simulink library "DBX_Control_lib"  (R2015a)
settings: Solver=ode45  SolverMode=SingleTasking  StartTime=0.0  StopTime=10.0  RelTol=1e-3
undefined symbols (not defined in the file or in its folder): a, A_M, C_d0, CG, h_1, h_2, h_3, kappa_Q, kappa_T, L_M, lambda_0_Q, lambda_0_T, m, Newton, Omega_TO, R, Raphson, rho, Rotation_sign, sigma, T_ctrl, theta_0, theta_1, Throtle_TO, Throtle_TTO_vec, v_i0, v_i_adim, Vx_adim, Vz_adim
undefined symbols (not defined in the file): hp_1, T_sim
libraries: DBX_Control_lib x15, simulink x8, vrlib x7, DBX_model x3, qcatlib x1, XXCopter_Control x1
(part 1 of 2)
settings Model: Creator=David  LastModifiedBy=David
settings OptimizationCC: BlockReduction=off  BooleanDataType=off
settings DebuggingCC: SaveWithParameterizedLinksMsg=none  UnderspecifiedInitializationDetection=Classic  MergeDetectMultiDrivingBlocksExec=none  SignalResolutionControl=TryResolveAllWithWarning  StrictBusMsg=Warning
settings HardwareCC: TargetUnknown=on

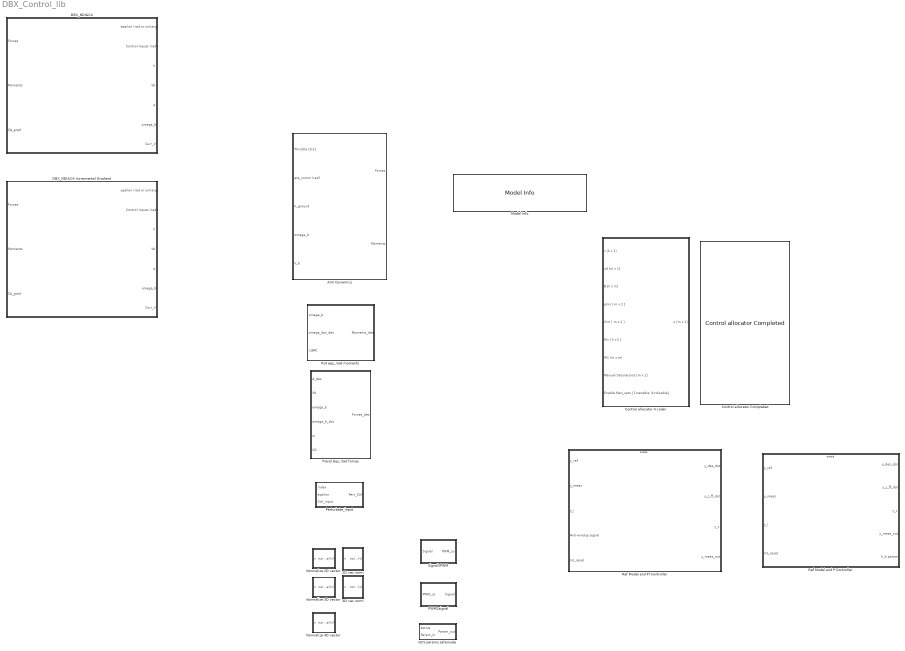
== system DBX_Control_lib ==
  2D vec norm : Subsystem  TreatAsAtomicUnit=on
  3D vec norm : Subsystem  TreatAsAtomicUnit=on
  Arm Dynamics : Subsystem  TreatAsAtomicUnit=on  mask(Arm dynamics, kinematics, forces and moments){arm_num=1, Rot_sign=Rotation_sign(1), Hub_pos=[1/3*L_M;-A_M/2;h_1], h_p=hp_1}
      mask prompts: arm_num "Arm number (1,2 or 3)"; Rot_sign "Rotation Sign"; Hub_pos "Hub position"; h_p "Hub to porpeller dist"
      mask help:
      | This block only accepts arms oriented in x-axis or y-axis: eta direction can only be [1,0,0] or [0,1,0]
      |
      | If Arm number 1 or  2 (Forward ones)
      | eta_dir==[0,1,0]
      |
      | If Arm number 3 (rear one)
      | eta_dir=[1,0,0]
      |
      | Usar SIEMPRE SI
      mask TypeOptions arm_num: Arms Kinematics DBX/Value
      mask TypeOptions Rot_sign: Aerodynamics Propeller DBX/Rot_signa
      mask TypeOptions Hub_pos: Arms Kinematics DBX/Hub_pos
      mask TypeOptions h_p: Arms Kinematics DBX/h_p
      mask DialogControl ParameterTabVar0 Prompt: Arm parameters
      mask Display: disp(['{\bf \fontsize{16}',sprintf('Arm number\n\n'),num2str(arm_num),sprintf('\n\n Dynamics '),'}'], 'texmode','on');
  Control allocator 4 coder : Subsystem  mask(Control allocator WLS){gamma=1e6, imax=100, T=T_sim}
      mask prompts: gamma "Weight of Control Error Cost (gamma)"; imax "Max # of iterations"; T "Sample Time"
      mask help:
      | Author: David Torres
      | Based on work of Ola Härkegård
  "Control allocator Completed " : qcatlib/Control allocator Completed   alg=WLS  CA_type=QP  iter_max=100  gamma=1  k_B=6  m_B=9  T=T_ctrl  tol=1e-5
  DBX_NDI&CA : Subsystem  TreatAsAtomicUnit=on
  DBX_NDI&CA Incremental Gradient : Subsystem  TreatAsAtomicUnit=on
  GCS params safemode : Subsystem  TreatAsAtomicUnit=on
  Model Info : simulink/Model-Wide Utilities/Model Info  Frame=on  DisplayStringWithTags=|  HorizontalTextAlignment=Center  LeftAlignmentValue=0.5  SourceBlockDiagram=DBX_Control_lib  TagMaxNumber=20
      | Model Info
      | 
      | Creado por %<Creator>
      | Modificado el %<LastModificationDate> por %<LastModifiedBy>
      | Version %<ModelVersion>
  Normalize 2D vector : Subsystem  TreatAsAtomicUnit=on
  Normalize 3D vector : Subsystem  TreatAsAtomicUnit=on
  Normalize 4D vector : Subsystem  TreatAsAtomicUnit=on
  PWM2signal : Subsystem  TreatAsAtomicUnit=on  mask{c=2100, a=900, d=1, b=0}
      mask prompts: c "PWM sup limit (us)"; a "PWM inf limit (us)"; d "Signal sup limit"; b "Signal inf limit"
      mask TypeOptions c: up_PWM/Value
      mask TypeOptions a: down_PWM/Value
      mask TypeOptions d: up_signal/Value
      mask TypeOptions b: down_signal/Value
  Perturbate_input : Subsystem
  Ref Model and P Controller : Subsystem  mask(Reference Model and Controller){tau=0.2, RisingSlewLimit=4, FallingSlewLimit=-4, K_f=1, K_b=1}
      mask prompts: tau "Desired time constant tau"; RisingSlewLimit "Reference max rising rate"; FallingSlewLimit "Reference max falling rate"; K_f "Rate Feedfordward Gain K_f"; K_b "Proportional Gain K_b"
      mask help:
      | Author: David Torres
      |
      | This block allows a design of the desired dynamics as a 1st order system and the controller of it with P and I actions, with feedforward in rate and anti-windup action.
      |
      |     Inputs: Signal reference, Signal measurement and anti-windup dignal.
      |     Outputs: Desired Signal rate
      |
      | The block shows the expected dynamics assuming the output is integrated with a PERFECT INTEGRATOR or an INTEGRATOR WITH DELAY(delta):
      |      NDI, CA and plant act as a perfect integrator or integrator with a delay delta.
      mask TypeOptions tau: Reference Model/tau
      mask TypeOptions RisingSlewLimit: Rate Limiter/RisingSlewLimit
      mask TypeOptions FallingSlewLimit: Rate Limiter/FallingSlewLimit
      mask TypeOptions K_f: K_f/Gain
      mask TypeOptions K_b: K_b params/Value
      mask Display:
      | K_ref=1/tau;
      | TF = tf([K_ref],[1 K_ref]);
      | 
      | [y,t]=step(TF);
      | S = stepinfo(y,t);
      | 
      | pos = get_param(gcb, 'Position');
      | width = pos(3) - pos(1);
      | height = pos(4) - pos(2);
      | t = t.*width/max(t);
      | y=y.*height/max(y);
      | plot(t,y);
      | S2 = stepinfo(y,t);
      | 
      | if S.Overshoot==0 % 1st order response
      |     text(S2.RiseTime ,height*0.85,['Rise time = ',num2str(S.RiseTime),'s' ]);
      |     text(S2.RiseTime ,height*0.75,['Settling Time = ',num2str(S.SettlingTime)]);
      | 
      | elseif S.Overshoot<0.05 % 2nd order response
      |     text(width*0.5 ,height*0.9,['Rise time = ',num2str(S.RiseTime),'s' ]);
      |     text(width*0.5 ,height*0.8,['Pike time = ',num2str(S.PeakTime),'s' ]);
      |     text(width*0.5 ,height*0.7,['Os = ',num2str(S.Peak)]);
      |     text(width*0.5 ,height*0.6,['SettlingTime = ',num2str(S.SettlingTime)]);
      | else % 2nd order response
      |     text(S2.PeakTime ,S2.Peak*0.85,['Peak time = ',num2str(S.PeakTime),'s' ]);
      |     text(S2.PeakTime ,S2.Peak*0.75,['Os = ',num2str(S.Peak)]);
      |     text(S2.PeakTime ,S2.Peak*0.65,['SettlingTime = ',num2str(S.SettlingTime)]);
      | end
      | 
      | 
      | [num,den] = tfdata(TF);
      | dpoly(num{:},den{:}, 's');
  Ref Model and PI Controller : Subsystem  mask(Reference Model and Controller){delta=0, tau=0.5, RisingSlewLimit=4, FallingSlewLimit=-4, K_f=1, K_a=1, Con_way=pro, omega_n=4, xi=0.5, Z1=-30, K_b=2*0.8*3, f_i=0.25*1/0.8^2, f_c=1}
      mask prompts: delta "Delay on assumed integration: delta (0 for ideal integration)"; tau "Desired time constant tau"; RisingSlewLimit "Reference max rising rate"; FallingSlewLimit "Reference max falling rate"; K_f "Rate Feedfordward Gain"; K_a "Anti-windup gain K_a"; Con_way "Expected response: Controller Design process"; omega_n "Desired 2nd order response omega_n"; xi "Desired 2nd order response  xi"; Z1 "Zero of controller"
      mask help:
      | Author: David Torres
      |
      | This block allows a design of the desired dynamics as a 1st order system and the controller of it with P and I actions, with feedforward in rate and anti-windup action.
      |
      |     Inputs: Signal reference, Signal measurement and anti-windup dignal.
      |     Outputs: Desired Signal rate
      |
      | The block shows the expected dynamics assuming the output is integrated with a PERFECT INTEGRATOR or an INTEGRATOR WITH DELAY(delta):
      |      NDI, CA and plant act as a perfect integrator or integrator with a delay delta.
      mask init:
      | val = get_param(gcb,'MaskValues');
      | 
      | K_ref=1/tau;	
      | % Controller design
      | switch lower(char(val{7}))
      |     case 'auto'
      |         K_b=2*xi*omega_n
      |         f_i=1/(4*xi^2)
      |         if f_i<0.25
      |             f_c = 0.5*(1+sqrt(1-4*f_i));
      |         else
      |             f_c = sqrt(f_i);
      |         end
      |         f_c
      |     case 'advanced'
      |         K_b=2*xi*omega_n;
      |         f_i=1/(4*xi^2);
      |         f_c =  -omega_n/(2*xi*Z1);  
      |     case 'pro'
      | end
      mask TypeOptions delta: PI Controller/delta
      mask TypeOptions tau: Reference Model/tau
      mask TypeOptions RisingSlewLimit: Rate Limiter/RisingSlewLimit
      mask TypeOptions FallingSlewLimit: Rate Limiter/FallingSlewLimit
      mask TypeOptions K_f: K_f/Gain
      mask TypeOptions K_a: PI Controller/K_a
      mask TypeOptions Con_way: auto | advanced | pro
      mask Callback Con_way:
      | val = get_param(gcb,'MaskValues');
      | switch lower(char(val{7}))
      |  case 'auto'
      |      set_param(gcb,'MaskVisibilities',{'on','on','on','on','on','on','on','on','on','off','off','off','off'});
      |  case 'advanced'
      |      set_param(gcb,'MaskVisibilities',{'on','on','on','on','on','on','on','on','on','on','off','off','off'});
      |  case 'pro'
      |      set_param(gcb,'MaskVisibilities',{'on','on','on','on','on','on','on','off','off','off','on','on','on'});
      |  end
      mask TypeOptions K_b: PI Controller/K_b
      mask TypeOptions f_i: PI Controller/f_i
      mask TypeOptions f_c: PI Controller/f_c
      mask Display:
      | RM = tf([K_ref],[1 K_ref]);
      | 
      | if delta==0
      |     TF_FF = tf([K_f K_b*f_c K_b*f_i*K_b],[1 K_b f_i*K_b^2]);
      | else
      |     s=tf('s');
      |     TF_FF = 1/(s+delta)*(K_f*s^2+K_b*(f_c*s+f_i*K_b))/(s + 1/(s+delta)*(K_b*s+f_i*K_b^2) );
      | end
      | TF = RM*TF_FF;
      | 
      | [y,t]=step(TF);
      | S = stepinfo(y,t);
      | 
      | pos = get_param(gcb, 'Position');
      | width = pos(3) - pos(1);
      | height = pos(4) - pos(2);
      | t = t.*width/max(t);
      | y=y.*height/max(y);
      | plot(t,y);
      | S2 = stepinfo(y,t);
      | 
      | if S.Overshoot==0 % 1st order response
      |     text(S2.RiseTime ,height*0.85,['Rise time = ',num2str(S.RiseTime),'s' ]);
      |     text(S2.RiseTime ,height*0.75,['Settling Time = ',num2str(S.SettlingTime)]);
      | 
      | elseif S.Overshoot<0.05 % 2nd order response
      |     text(width*0.5 ,height*0.9,['Rise time = ',num2str(S.RiseTime),'s' ]);
      |     text(width*0.5 ,height*0.8,['Pike time = ',num2str(S.PeakTime),'s' ]);
      |     text(width*0.5 ,height*0.7,['Os = ',num2str(S.Peak)]);
      |     text(width*0.5 ,height*0.6,['SettlingTime = ',num2str(S.SettlingTime)]);
      | else % 2nd order response
      |     text(S2.PeakTime ,S2.Peak*0.85,['Peak time = ',num2str(S.PeakTime),'s' ]);
      |     text(S2.PeakTime ,S2.Peak*0.75,['Os = ',num2str(S.Peak)]);
      |     text(S2.PeakTime ,S2.Peak*0.65,['SettlingTime = ',num2str(S.SettlingTime)]);
      | end
      | 
      | text(0.1*width,0.1*height,['EXPECTED CLOSED-LOOP RESPONSE: INTEGRATION DELAY OF ',num2str(delta),'s ']);
      | 
      | [num,den] = tfdata(TF);
      | dpoly(num{:},den{:}, 's');
  Rot eqs_ Get moments : Subsystem  TreatAsAtomicUnit=on
  Signal2PWM : Subsystem  TreatAsAtomicUnit=on  mask{b=1, d=0, a=2100, c=900}
      mask prompts: b "Signal sup limit"; d "Signal inf limit"; a "PWM sup limit (us)"; c "PWM inf limit (us)"
      mask TypeOptions b: up_signal/Value
      mask TypeOptions d: down_signal/Value
      mask TypeOptions a: up_PWM/Value
      mask TypeOptions c: down_PWM/Value
  Transl Eqs_ Get forces : Subsystem  TreatAsAtomicUnit=on

== system DBX_Control_lib/2D vec norm ==
  v : Inport
  norm^2rm : Subsystem  TreatAsAtomicUnit=on
  sqrt : Sqrt  AlgorithmType=Newton-Raphson  SaturateOnIntegerOverflow=on
  norm(v) : Outport
  wires:
  sqrt/1 -> norm(v)/1
  norm^2rm/1(norm(v)) -> sqrt/1
  v/1 -> norm^2rm/1(v)

== system DBX_Control_lib/3D vec norm ==
  v : Inport
  norm^2rm : Subsystem  TreatAsAtomicUnit=on
  sqrt : Sqrt  AlgorithmType=Newton-Raphson  SaturateOnIntegerOverflow=on
  norm(v) : Outport
  wires:
  v/1 -> norm^2rm/1(v)
  norm^2rm/1(norm(v)) -> sqrt/1
  sqrt/1 -> norm(v)/1

== system DBX_Control_lib/Arm Dynamics ==
  note: Angulo del brazo
  Throttle [0-1] : Inport
  eta_comm (rad) : Inport  Port=2
  h_ground : Inport  Port=3
  omega_b : Inport  Port=4
  V_b : Inport  Port=5
  Aerodynamics Propeller DBX : Subsystem  TreatAsAtomicUnit=on  mask{Rot_signa=Rot_sign}
      mask prompts: Rot_signa "Rotation Sign"
      settings: MinAlgLoopOccurrences=on
      mask TypeOptions Rot_signa: Rotation_sign/Value
  Arms Kinematics DBX : Subsystem  TreatAsAtomicUnit=on  mask{Value=arm_num, Hub_pos=Hub_pos, h_p=h_p}
      mask prompts: Value "Arm number (1,2 or 3)"; Hub_pos "Hub position"; h_p "Hub to porpeller dist"
      mask TypeOptions Value: Arm_no/Value
      mask TypeOptions Hub_pos: Hub_position aka r_RP_i/Value
      mask TypeOptions h_p: h_p_i/Value
  Cross Product : vrlib/Utilities/Cross Product
  "ESC+Motor Dynamcis " : Subsystem  TreatAsAtomicUnit=on  VariantControl=Variant_completed
  F_b->F_A : Product  Multiplication=Matrix(*)
  Permute Dimensions : PermuteDimensions
  V^A (m/s) : Sum
  Forces : Outport
  Moments : Outport  Port=2
  wires:
  "ESC+Motor Dynamcis "/1(Omega_out) -> Aerodynamics Propeller DBX/1(Omega)
  Permute Dimensions/1 -> F_b->F_A/1
  V^A (m/s)/1 -> F_b->F_A/2
  eta_comm (rad)/1 -> Arms Kinematics DBX/1(eta (rad))
  Aerodynamics Propeller DBX/2(Moments_prop @Fb) -> Moments/1
  Aerodynamics Propeller DBX/1(Forces_prop @Fb) -> Forces/1
  Arms Kinematics DBX/1(r_p (m)) -> Cross Product/2, Aerodynamics Propeller DBX/3(r_p)
  Arms Kinematics DBX/2(T_F_a,Fb) -> Permute Dimensions/1, Aerodynamics Propeller DBX/5(T_FaFb)
  F_b->F_A/1 -> Aerodynamics Propeller DBX/4(V^A)
  V_b/1 -> V^A (m/s)/1
  Cross Product/1 -> V^A (m/s)/2
  omega_b/1 -> Cross Product/1
  h_ground/1 -> Aerodynamics Propeller DBX/2(h_ground)
  Throttle [0-1]/1 -> "ESC+Motor Dynamcis "/1(Throttle)

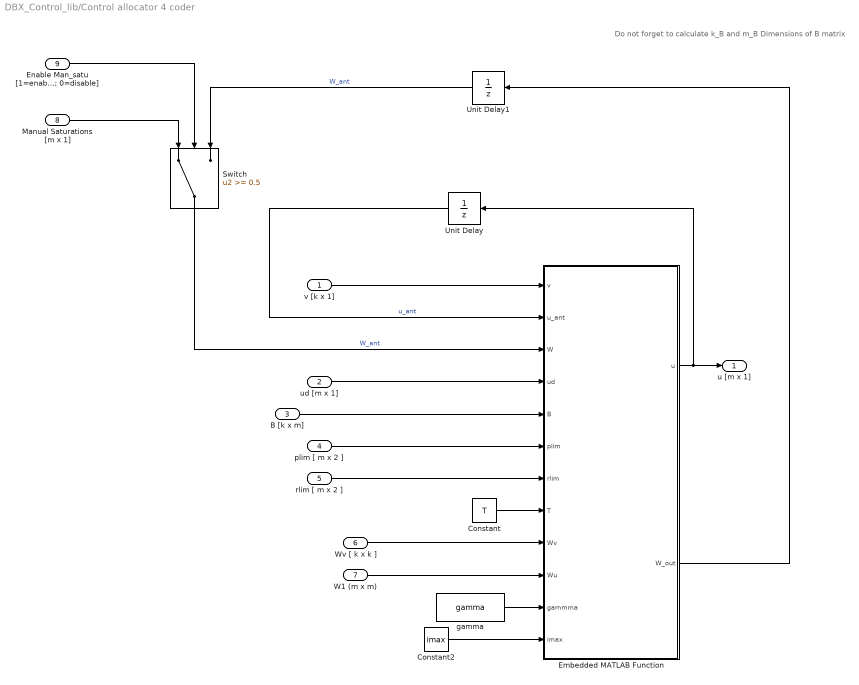
== system DBX_Control_lib/Control allocator 4 coder ==
  note: Do not forget to calculate k_B and m_B Dimensions of B matrix
  v [k x 1] : Inport
  ud [m x 1] : Inport  Port=2
  B [k x m] : Inport  Port=3
  plim [ m x 2 ] : Inport  Port=4
  rlim [ m x 2 ] : Inport  Port=5
  Wv [ k x k ] : Inport  Port=6
  W1 (m x m) : Inport  Port=7
  Manual Saturations [m x 1] : Inport  Port=8
  Enable Man_satu [1=enable; 0=disable] : Inport  Port=9
  Constant : Constant  Value=T  OutDataTypeStr=single
  Constant2 : Constant  Value=imax  OutDataTypeStr=single
  Embedded MATLAB Function : MATLAB Function  TreatAsAtomicUnit=on
  Switch : Switch  Threshold=0.5  SampleTime=T
  Unit Delay : UnitDelay  InitialCondition=zeros(9,1)  SampleTime=T
  Unit Delay1 : UnitDelay  InitialCondition=zeros(9,1)  SampleTime=T
  gamma : Constant  Value=gamma  OutDataTypeStr=single
  u [m x 1] : Outport
  wires:
  Enable Man_satu [1=enable; 0=disable]/1 -> Switch/2
  Manual Saturations [m x 1]/1 -> Switch/1
  Unit Delay1/1 -> Switch/3  "W_ant"
  Embedded MATLAB Function/1(u) -> Unit Delay/1, u [m x 1]/1
  Switch/1 -> Embedded MATLAB Function/3(W)  "W_ant"
  Embedded MATLAB Function/2(W_out) -> Unit Delay1/1
  ud [m x 1]/1 -> Embedded MATLAB Function/4(ud)
  W1 (m x m)/1 -> Embedded MATLAB Function/10(Wu)
  Wv [ k x k ]/1 -> Embedded MATLAB Function/9(Wv)
  rlim [ m x 2 ]/1 -> Embedded MATLAB Function/7(rlim)
  plim [ m x 2 ]/1 -> Embedded MATLAB Function/6(plim)
  B [k x m]/1 -> Embedded MATLAB Function/5(B)
  Unit Delay/1 -> Embedded MATLAB Function/2(u_ant)  "u_ant"
  v [k x 1]/1 -> Embedded MATLAB Function/1(v)
  Constant/1 -> Embedded MATLAB Function/8(T)
  gamma/1 -> Embedded MATLAB Function/11(gammma)
  Constant2/1 -> Embedded MATLAB Function/12(imax)

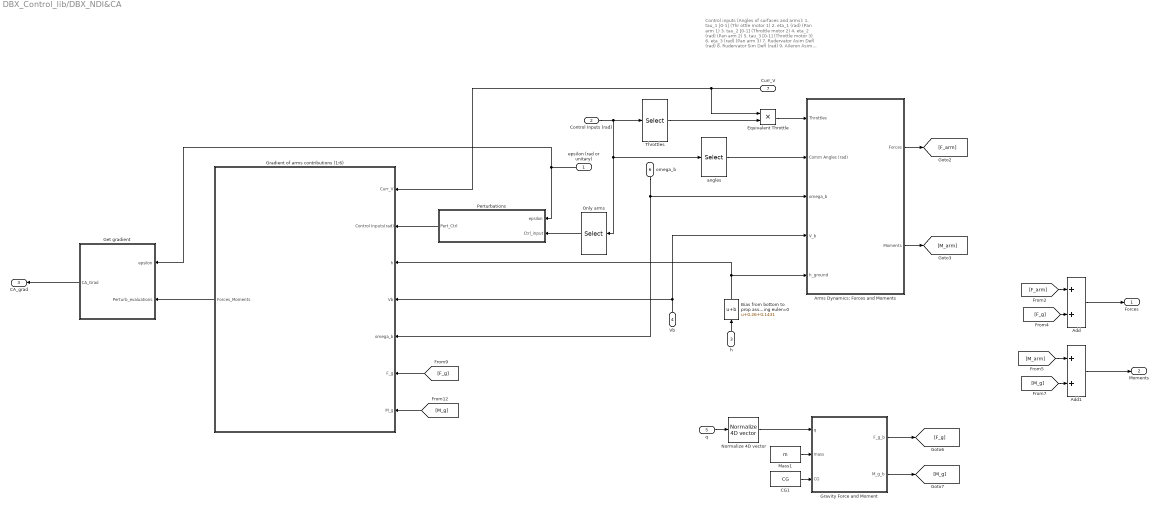
== system DBX_Control_lib/DBX_NDI&CA ==
  note: Control inputs (Angles  of surfaces and arms):
      |
      | 1. tau_1 [0-1] (Thr ottle motor 1)
      | 2. eta_1 (rad)  (Pan arm 1)
      |
      | 3. tau_2 [0-1] (Throttle motor 2)
      | 4. eta_2 (rad)  (Pan arm 2)
      |
      | 5. tau_3 [0-1] (Throttle motor 3)
      | 6. eta_3 (rad)  (Pan arm  3)
      |
      | 7. Rudervator Asim Defl (rad)
      | 8. Rudervator Sim Defl (rad)
      | 9. Aileron Asim Defl (rad)
  "epsilon (rad or unitary) " : Inport
  Control Inputs (rad) : Inport  Port=2
  h : Inport  Port=3
  Vb : Inport  Port=4
  q : Inport  Port=5
  omega_b : Inport  Port=6
  Curr_V : Inport  Port=7
  Add : Sum
  Add1 : Sum
  Arms Dynamics: Forces and Moments : Subsystem  TreatAsAtomicUnit=on
  Bias from bottom to prop assuming euler=0 : Bias  Bias=0.26+0.1431
  CG1 : Constant  Value=CG
  Equivalent Throttle : Product  Inputs=**
  Get gradient : MATLAB Function  TreatAsAtomicUnit=on
  Gradient of arms contributions (1:6) : Subsystem  TreatAsAtomicUnit=on
  Gravity Force and Moment : MATLAB Function  TreatAsAtomicUnit=on
  Mass1 : Constant  Value=m
  Normalize 4D vector : DBX_Control_lib/Normalize 4D vector
  Only arms : Selector  InputPortWidth=9  Indices=[1:6]
  Perturbations : MATLAB Function  TreatAsAtomicUnit=on
  Throttles : Selector  InputPortWidth=9  Indices=[1,3,5]
  "angles " : Selector  InputPortWidth=9  Indices=[2,4,6]
  Forces : Outport
  Moments : Outport  Port=2
  CA_grad : Outport  Port=3
  wires:
  Only arms/1 -> Perturbations/2(Ctrl_input)
  CG1/1 -> Gravity Force and Moment/3(CG)
  Gravity Force and Moment/1(F_g_b) -> [F_g]
  h/1 -> Bias from bottom to prop assuming euler=0/1
  q/1 -> Normalize 4D vector/1
  Bias from bottom to prop assuming euler=0/1 -> Arms Dynamics: Forces and Moments/5(h_ground), Gradient of arms contributions (1:6)/3(h)
  "angles "/1 -> Arms Dynamics: Forces and Moments/2(Comm Angles (rad))
  Vb/1 -> Gradient of arms contributions (1:6)/4(Vb), Arms Dynamics: Forces and Moments/4(V_b)
  omega_b/1 -> Arms Dynamics: Forces and Moments/3(omega_b), Gradient of arms contributions (1:6)/5(omega_b)
  Mass1/1 -> Gravity Force and Moment/2(mass)
  Arms Dynamics: Forces and Moments/1(Forces) -> [F_arm]
  Arms Dynamics: Forces and Moments/2(Moments) -> [M_arm]
  Gravity Force and Moment/2(M_g_b) -> [M_g]
  [F_arm] -> Add/1
  [F_g] -> Add/2
  [M_arm] -> Add1/1
  [M_g] -> Add1/2
  Throttles/1 -> Equivalent Throttle/2
  Control Inputs (rad)/1 -> Only arms/1, "angles "/1, Throttles/1
  Add/1 -> Forces/1
  Equivalent Throttle/1 -> Arms Dynamics: Forces and Moments/1(Throttles)
  Curr_V/1 -> Equivalent Throttle/1, Gradient of arms contributions (1:6)/1(Curr_V)
  Add1/1 -> Moments/1
  Normalize 4D vector/1 -> Gravity Force and Moment/1(q)
  [M_g] -> Gradient of arms contributions (1:6)/7(M_g)
  [F_g] -> Gradient of arms contributions (1:6)/6(F_g)
  Gradient of arms contributions (1:6)/1(Forces_Moments) -> Get gradient/2(Perturb_evaluations)
  Perturbations/1(Pert_Ctrl) -> Gradient of arms contributions (1:6)/2("Control Inputs(rad) ")
  "epsilon (rad or unitary) "/1 -> Get gradient/1(epsilon), Perturbations/1(epsilon)
  Get gradient/1(CA_Grad) -> CA_grad/1

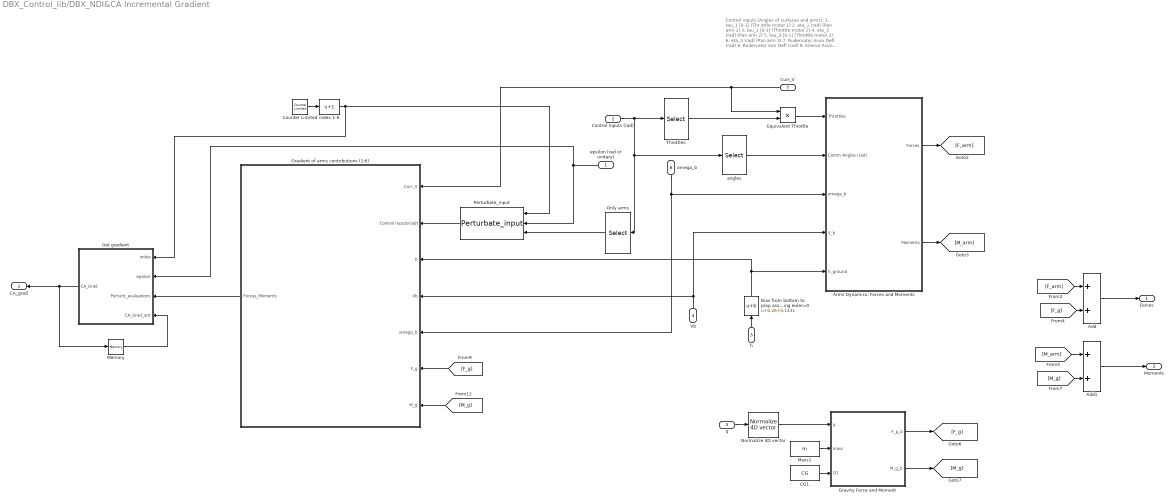
== system DBX_Control_lib/DBX_NDI&CA Incremental Gradient ==
  note: Control inputs (Angles  of surfaces and arms):
      |
      | 1. tau_1 [0-1] (Thr ottle motor 1)
      | 2. eta_1 (rad)  (Pan arm 1)
      |
      | 3. tau_2 [0-1] (Throttle motor 2)
      | 4. eta_2 (rad)  (Pan arm 2)
      |
      | 5. tau_3 [0-1] (Throttle motor 3)
      | 6. eta_3 (rad)  (Pan arm  3)
      |
      | 7. Rudervator Asim Defl (rad)
      | 8. Rudervator Sim Defl (rad)
      | 9. Aileron Asim Defl (rad)
  "epsilon (rad or unitary) " : Inport
  Control Inputs (rad) : Inport  Port=2
  h : Inport  Port=3
  Vb : Inport  Port=4
  q : Inport  Port=5
  omega_b : Inport  Port=6
  Curr_V : Inport  Port=7
  Add : Sum
  Add1 : Sum
  Arms Dynamics: Forces and Moments : Subsystem  TreatAsAtomicUnit=on
  Bias from bottom to prop assuming euler=0 : Bias  Bias=0.26+0.1431
  CG1 : Constant  Value=CG  OutDataTypeStr=single
  Counter Limited : simulink/Sources/Counter Limited  uplimit=5  tsamp=T_ctrl
  Equivalent Throttle : Product  Inputs=**
  Get gradient : MATLAB Function  TreatAsAtomicUnit=on
  Gradient of arms contributions (1:6) : Subsystem  TreatAsAtomicUnit=on
  Gravity Force and Moment : MATLAB Function  TreatAsAtomicUnit=on
  Mass1 : Constant  Value=m  OutDataTypeStr=single
  Memory : Memory  X0=zeros(6,9)  InheritSampleTime=on
  Normalize 4D vector : DBX_Control_lib/Normalize 4D vector
  Only arms : Selector  InputPortWidth=9  Indices=[1:6]
  Perturbate_input : DBX_Control_lib/Perturbate_input
  Throttles : Selector  InputPortWidth=9  Indices=[1,3,5]
  "angles " : Selector  InputPortWidth=9  Indices=[2,4,6]
  index 1-6 : Bias  Bias=1
  Forces : Outport
  Moments : Outport  Port=2
  CA_grad : Outport  Port=3
  wires:
  Only arms/1 -> Perturbate_input/3
  CG1/1 -> Gravity Force and Moment/3(CG)
  Gravity Force and Moment/1(F_g_b) -> [F_g]
  h/1 -> Bias from bottom to prop assuming euler=0/1
  q/1 -> Normalize 4D vector/1
  Bias from bottom to prop assuming euler=0/1 -> Arms Dynamics: Forces and Moments/5(h_ground), Gradient of arms contributions (1:6)/3(h)
  "angles "/1 -> Arms Dynamics: Forces and Moments/2(Comm Angles (rad))
  Vb/1 -> Gradient of arms contributions (1:6)/4(Vb), Arms Dynamics: Forces and Moments/4(V_b)
  omega_b/1 -> Arms Dynamics: Forces and Moments/3(omega_b), Gradient of arms contributions (1:6)/5(omega_b)
  Mass1/1 -> Gravity Force and Moment/2(mass)
  Arms Dynamics: Forces and Moments/1(Forces) -> [F_arm]
  Arms Dynamics: Forces and Moments/2(Moments) -> [M_arm]
  Gravity Force and Moment/2(M_g_b) -> [M_g]
  [F_arm] -> Add/1
  [F_g] -> Add/2
  [M_arm] -> Add1/1
  [M_g] -> Add1/2
  Throttles/1 -> Equivalent Throttle/2
  Control Inputs (rad)/1 -> Only arms/1, "angles "/1, Throttles/1
  Add/1 -> Forces/1
  Equivalent Throttle/1 -> Arms Dynamics: Forces and Moments/1(Throttles)
  Curr_V/1 -> Equivalent Throttle/1, Gradient of arms contributions (1:6)/1(Curr_V)
  Add1/1 -> Moments/1
  Normalize 4D vector/1 -> Gravity Force and Moment/1(q)
  [M_g] -> Gradient of arms contributions (1:6)/7(M_g)
  [F_g] -> Gradient of arms contributions (1:6)/6(F_g)
  Gradient of arms contributions (1:6)/1(Forces_Moments) -> Get gradient/3(Perturb_evaluations)
  Perturbate_input/1 -> Gradient of arms contributions (1:6)/2("Control Inputs(rad) ")
  "epsilon (rad or unitary) "/1 -> Perturbate_input/2, Get gradient/2(epsilon)
  Get gradient/1(CA_Grad) -> CA_grad/1, Memory/1
  Counter Limited/1 -> index 1-6/1
  index 1-6/1 -> Perturbate_input/1, Get gradient/1(index)
  Memory/1 -> Get gradient/4(CA_Grad_ant)

== system DBX_Control_lib/GCS params safemode ==
  Active : Inport
  Param_in : Inport  Port=2
  Data Type Conversion : DataTypeConversion  OutDataTypeStr=boolean
  Delay : Delay  DelayLength=5  InitialCondition=0
  Logical Operator : Logic  IconShape=distinctive  AllPortsSameDT=off  OutDataTypeStr=boolean
  Relational Operator : RelationalOperator  Operator=~=  OutDataTypeStr=boolean
  Sample&Hold : Subsystem  TreatAsAtomicUnit=on
  Unit Delay : UnitDelay  SampleTime=-1
  Param_out : Outport
  wires:
  Param_in/1 -> Sample&Hold/1(In1), Relational Operator/1, Unit Delay/1
  Unit Delay/1 -> Relational Operator/2
  Relational Operator/1 -> Logical Operator/2
  Active/1 -> Delay/1
  Data Type Conversion/1 -> Logical Operator/1
  Logical Operator/1 -> Sample&Hold/Trigger
  Sample&Hold/1(Out1) -> Param_out/1
  Delay/1 -> Data Type Conversion/1

== system DBX_Control_lib/Normalize 2D vector ==
  v : Inport
  Bias : Bias  Bias=eps
  Demux : Demux  Outputs=2
  Dot Product : DotProduct  InputSameDT=on  OutDataTypeStr=Inherit: Inherit via internal rule
  Math Function : Math  Operator=reciprocal  SaturateOnIntegerOverflow=on
  Mux : Mux  Inputs=2
  Product2 : Product  Inputs=**
  Product3 : Product  Inputs=**
  Sqrt : Sqrt  SaturateOnIntegerOverflow=on
  normal(v) : Outport
  wires:
  Math Function/1 -> Product2/2, Product3/2
  Demux/2 -> Product3/1
  Demux/1 -> Product2/1
  Mux/1 -> normal(v)/1
  v/1 -> Dot Product/2, Dot Product/1, Demux/1
  Bias/1 -> Math Function/1
  Product2/1 -> Mux/1
  Product3/1 -> Mux/2
  Dot Product/1 -> Sqrt/1
  Sqrt/1 -> Bias/1

== system DBX_Control_lib/Normalize 3D vector ==
  v : Inport
  3D vec norm : XXCopter_Control/3D vec norm
  Bias : Bias  Bias=eps
  Demux : Demux  Outputs=3
  Math Function : Math  Operator=reciprocal  SaturateOnIntegerOverflow=on
  Mux : Mux  Inputs=3
  Product1 : Product  Inputs=**
  Product2 : Product  Inputs=**
  Product3 : Product  Inputs=**
  normal(v) : Outport
  wires:
  Demux/2 -> Product3/1
  Demux/1 -> Product2/1
  Mux/1 -> normal(v)/1
  v/1 -> 3D vec norm/1, Demux/1
  3D vec norm/1 -> Bias/1
  Product2/1 -> Mux/1
  Product3/1 -> Mux/2
  Demux/3 -> Product1/1
  Math Function/1 -> Product2/2, Product3/2, Product1/2
  Product1/1 -> Mux/3
  Bias/1 -> Math Function/1

== system DBX_Control_lib/Normalize 4D vector ==
  v : Inport
  4D vec norm : Subsystem  TreatAsAtomicUnit=on
  Bias : Bias  Bias=eps
  Demux : Demux
  Math Function : Math  Operator=reciprocal  SaturateOnIntegerOverflow=on
  Mux : Mux
  Product{1..4} (4 alike) : Product  Inputs=**
  normal(v) : Outport
  wires:
  Bias/1 -> Math Function/1
  Product1/1 -> Mux/3
  Math Function/1 -> Product4/2, Product1/2, Product3/2, Product2/2
  Demux/3 -> Product1/1
  Product3/1 -> Mux/2
  Product2/1 -> Mux/1
  4D vec norm/1(norm(v)) -> Bias/1
  v/1 -> 4D vec norm/1(v), Demux/1
  Mux/1 -> normal(v)/1
  Demux/1 -> Product2/1
  Demux/2 -> Product3/1
  Demux/4 -> Product4/1
  Product4/1 -> Mux/4

== system DBX_Control_lib/PWM2signal ==
  PWM_us : Inport
  Add : Sum  Inputs=+-
  Add1 : Sum  Inputs=+-
  Add2 : Sum  Inputs=+-
  Add3 : Sum
  Divide : Product  Inputs=*/
  Divide1 : Product  Inputs=**
  down_PWM : Constant  Value=a
  down_signal : Constant  Value=b
  up_PWM : Constant  Value=c
  up_signal : Constant  Value=d
  Signal : Outport
  wires:
  Add3/1 -> Signal/1
  Divide1/1 -> Add3/2
  Add2/1 -> Divide1/1
  Divide/1 -> Divide1/2
  down_signal/1 -> Add2/2, Add3/1
  up_signal/1 -> Add2/1
  Add/1 -> Divide/1
  Add1/1 -> Divide/2
  up_PWM/1 -> Add1/1
  down_PWM/1 -> Add1/2, Add/2
  PWM_us/1 -> Add/1

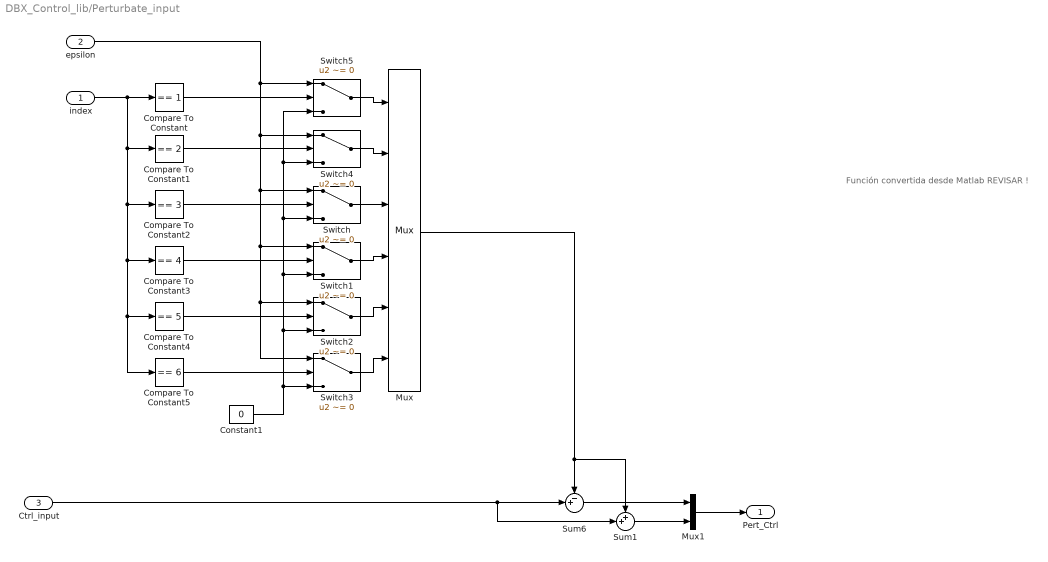
== system DBX_Control_lib/Perturbate_input ==
  note: Función convertida desde Matlab
      | REVISAR !
  index : Inport
  epsilon : Inport  Port=2
  Ctrl_input : Inport  Port=3
  Compare To Constant : simulink/Logic and Bit Operations/Compare To Constant  relop===  const=1  OutDataTypeStr=boolean
  Compare To Constant1 : simulink/Logic and Bit Operations/Compare To Constant  relop===  const=2  OutDataTypeStr=boolean
  Compare To Constant2 : simulink/Logic and Bit Operations/Compare To Constant  relop===  const=3  OutDataTypeStr=boolean
  Compare To Constant3 : simulink/Logic and Bit Operations/Compare To Constant  relop===  const=4  OutDataTypeStr=boolean
  Compare To Constant4 : simulink/Logic and Bit Operations/Compare To Constant  relop===  const=5  OutDataTypeStr=boolean
  Compare To Constant5 : simulink/Logic and Bit Operations/Compare To Constant  relop===  const=6  OutDataTypeStr=boolean
  Constant1 : Constant  Value=0  OutDataTypeStr=single
  Mux : Mux  Inputs=6
  Mux1 : Mux  Inputs=2
  Sum1 : Sum  Inputs=++|
  Sum6 : Sum  Inputs=-+|
  Switch{,1..5} (6 alike) : Switch  Criteria=u2 ~= 0
  Pert_Ctrl : Outport
  wires:
  Mux1/1 -> Pert_Ctrl/1
  Constant1/1 -> Switch2/3, Switch1/3, Switch/3, Switch4/3, Switch5/3, Switch3/3
  epsilon/1 -> Switch5/1, Switch4/1, Switch/1, Switch1/1, Switch2/1, Switch3/1
  index/1 -> Compare To Constant5/1, Compare To Constant4/1, Compare To Constant3/1, Compare To Constant2/1, Compare To Constant1/1, Compare To Constant/1
  Compare To Constant/1 -> Switch5/2
  Compare To Constant1/1 -> Switch4/2
  Compare To Constant2/1 -> Switch/2
  Compare To Constant3/1 -> Switch1/2
  Compare To Constant4/1 -> Switch2/2
  Compare To Constant5/1 -> Switch3/2
  Switch5/1 -> Mux/1
  Switch4/1 -> Mux/2
  Switch/1 -> Mux/3
  Switch1/1 -> Mux/4
  Switch2/1 -> Mux/5
  Switch3/1 -> Mux/6
  Ctrl_input/1 -> Sum1/2, Sum6/2
  Mux/1 -> Sum1/1, Sum6/1
  Sum6/1 -> Mux1/1
  Sum1/1 -> Mux1/2

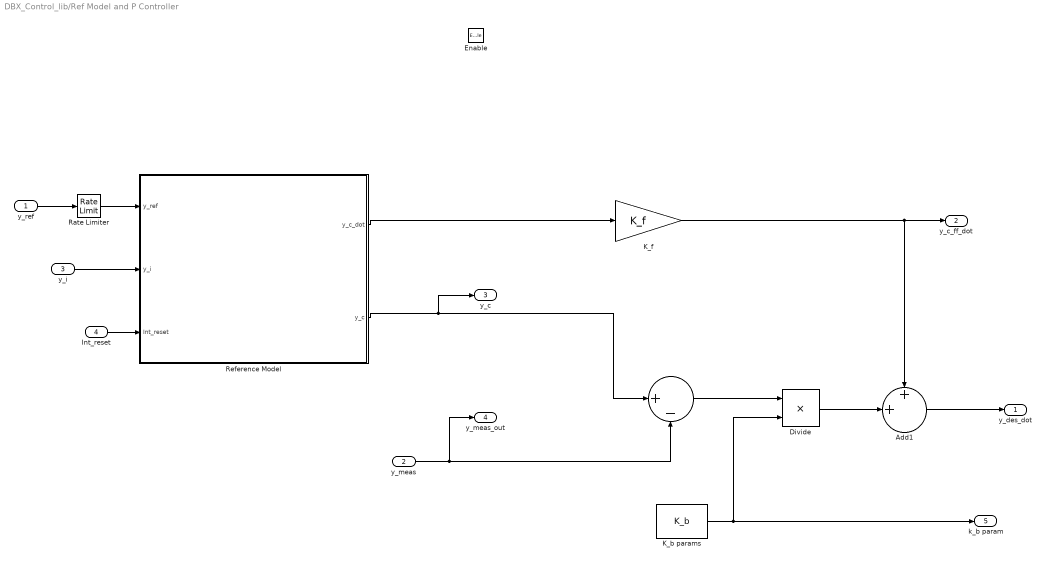
== system DBX_Control_lib/Ref Model and P Controller ==
  y_ref : Inport
  y_meas : Inport  Port=2
  y_i : Inport  Port=3
  Int_reset : Inport  Port=4
  Enable : EnablePort  StatesWhenEnabling=reset
  " " : Sum  Inputs=|+-
  Add1 : Sum  Inputs=++|
  Divide : Product  Inputs=**
  K_b params : Constant  Value=K_b  OutDataTypeStr=single
  K_f : Gain  Gain=K_f
  Rate Limiter : RateLimiter  RisingSlewLimit=RisingSlewLimit  FallingSlewLimit=FallingSlewLimit  SampleTimeMode=inherited
  Reference Model : Subsystem  mask{tau=tau}
      mask prompts: tau "1st order time constant (tau)"
      mask init:
      | K_ref=1/tau;
      mask TypeOptions tau: tau/Value
      mask Display:
      | [y,t]=step(tf([K_ref],[1 K_ref]));
      | pos = get_param(gcb, 'Position');
      | width = pos(3) - pos(1);
      | height = pos(4) - pos(2);
      | t = t.*width/max(t);
      | y=y.*height/max(y);
      | plot(t,y);
      | 
      | 
      | text(0.5*width,0.92*height,['tau=',num2str(tau)]);
      | 
      | dpoly([K_ref],[1 K_ref], 's')
  y_des_dot : Outport
  y_c_ff_dot : Outport  Port=2
  y_c : Outport  Port=3
  y_meas_out : Outport  Port=4
  k_b param : Outport  Port=5
  wires:
  Divide/1 -> Add1/2
  K_f/1 -> Add1/1, y_c_ff_dot/1
  Reference Model/1(y_c_dot) -> K_f/1
  Add1/1 -> y_des_dot/1
  y_ref/1 -> Rate Limiter/1
  " "/1 -> Divide/1
  Reference Model/2(y_c) -> " "/1, y_c/1
  y_meas/1 -> " "/2, y_meas_out/1
  K_b params/1 -> Divide/2, k_b param/1
  y_i/1 -> Reference Model/2(y_i)
  Rate Limiter/1 -> Reference Model/1(y_ref)
  Int_reset/1 -> Reference Model/3(Int_reset)

== system DBX_Control_lib/Ref Model and PI Controller ==
  y_ref : Inport
  y_meas : Inport  Port=2
  y_i : Inport  Port=3
  Anti-windup signal : Inport  Port=4
  Int_reset : Inport  Port=5
  Enable : EnablePort  StatesWhenEnabling=reset
  Add1 : Sum  Inputs=++|
  K_f : Gain  Gain=K_f
  PI Controller : Subsystem  mask{K_b=K_b, f_i=f_i, f_c=f_c, K_a=K_a, delta=delta}
      mask prompts: K_b "K_b proportional term"; f_i "f_i integral term"; f_c "f_c fedfordward term"; K_a "Anti-windup gain"; delta "Integrator delay"
      mask TypeOptions K_b:
      | K_b/Gain | K_b
      | /Value
      mask TypeOptions f_i: f_i/Value
      mask TypeOptions f_c: f_c/Gain
      mask TypeOptions K_a: K_a/Gain
      mask Display:
      | if delta==0
      |     TF = tf(K_b*[f_c f_i*K_b],[1 K_b f_i*K_b^2]);
      | else
      |     s=tf('s');
      |     TF = 1/(s+delta)*K_b*(f_c*s+f_i*K_b)/(s*( 1+1/(s+delta)*K_b ) + 1/(s+delta)*f_i*K_b^2 );
      | end
      | 
      | [y,t]=step(TF);
      | S = stepinfo(y,t);
      | 
      | pos = get_param(gcb, 'Position');
      | width = pos(3) - pos(1);
      | height = pos(4) - pos(2);
      | t = t.*width/max(t);
      | y=y.*height/max(y);
      | plot(t,y);
      | 
      | S2 = stepinfo(y,t);
      | text(S2.PeakTime ,S2.Peak*0.85,['Peak time = ',num2str(S.PeakTime),'s' ]);
      | text(S2.PeakTime ,S2.Peak*0.75,['Os = ',num2str(S.Peak)]);
      | text(S2.PeakTime ,S2.Peak*0.75,['Os = ',num2str(S.Peak)]);
      | text(S2.PeakTime ,S2.Peak*0.65,['SettlingTime = ',num2str(S.SettlingTime)]);
      | 
      | text(0.1*width,0.1*height,['EXPECTED CLOSED-LOOP RESPONSE: INTEGRATION DELAY OF ',num2str(delta),'s ']);
      | 
      | [num,den] = tfdata(TF);
      | dpoly(num{:},den{:}, 's');
  Rate Limiter : RateLimiter  RisingSlewLimit=RisingSlewLimit  FallingSlewLimit=FallingSlewLimit  SampleTimeMode=inherited
  Reference Model : Subsystem  mask{tau=tau}
      mask prompts: tau "1st order time constant (tau)"
      mask init:
      | K_ref=1/tau;
      mask TypeOptions tau: tau/Value
      mask Display:
      | [y,t]=step(tf([K_ref],[1 K_ref]));
      | pos = get_param(gcb, 'Position');
      | width = pos(3) - pos(1);
      | height = pos(4) - pos(2);
      | t = t.*width/max(t);
      | y=y.*height/max(y);
      | plot(t,y);
      | 
      | 
      | text(0.5*width,0.92*height,['tau=',num2str(tau)]);
      | 
      | dpoly([K_ref],[1 K_ref], 's')
  y_des_dot : Outport
  y_c_ff_dot : Outport  Port=2
  y_c : Outport  Port=3
  y_meas_out : Outport  Port=4
  wires:
  y_ref/1 -> Rate Limiter/1
  Reference Model/2(y_c) -> PI Controller/1(y_c), y_c/1
  Add1/1 -> y_des_dot/1
  Reference Model/1(y_c_dot) -> K_f/1
  K_f/1 -> y_c_ff_dot/1, Add1/1
  PI Controller/1(y_des_dot) -> Add1/2
  Anti-windup signal/1 -> PI Controller/3(Anti-windup signal)
  y_meas/1 -> y_meas_out/1, PI Controller/2(y_meas)
  y_i/1 -> Reference Model/2(y_i)
  Rate Limiter/1 -> Reference Model/1(y_ref)
  Int_reset/1 -> PI Controller/4(Int_reset), Reference Model/3(Int_reset)

== system DBX_Control_lib/Rot eqs_ Get moments ==
  omega_b : Inport
  omega_dot_des : Inport  Port=2
  I_BAC : Inport  Port=3
  Cross Product : vrlib/Utilities/Cross Product
  Matrix Multiply : Product  Multiplication=Matrix(*)
  Matrix Multiply1 : Product  Multiplication=Matrix(*)
  Moment des : Sum
  Moments_des : Outport
  wires:
  Cross Product/1 -> Moment des/1
  Matrix Multiply/1 -> Cross Product/2
  omega_b/1 -> Matrix Multiply/2, Cross Product/1
  I_BAC/1 -> Matrix Multiply1/1, Matrix Multiply/1
  omega_dot_des/1 -> Matrix Multiply1/2
  Matrix Multiply1/1 -> Moment des/2
  Moment des/1 -> Moments_des/1

== system DBX_Control_lib/Signal2PWM ==
  Signal : Inport
  Add : Sum  Inputs=+-
  Add1 : Sum  Inputs=+-
  Add2 : Sum  Inputs=+-
  Add3 : Sum
  Divide : Product  Inputs=*/
  Divide1 : Product  Inputs=**
  down_PWM : Constant  Value=c  OutDataTypeStr=single
  down_signal : Constant  Value=d  OutDataTypeStr=single
  up_PWM : Constant  Value=a  OutDataTypeStr=single
  up_signal : Constant  Value=b  OutDataTypeStr=single
  PWM_us : Outport
  wires:
  Signal/1 -> Add/1
  down_signal/1 -> Add/2, Add1/2
  up_signal/1 -> Add1/1
  Add1/1 -> Divide/2
  Add/1 -> Divide/1
  up_PWM/1 -> Add2/1
  down_PWM/1 -> Add3/1, Add2/2
  Divide/1 -> Divide1/2
  Add2/1 -> Divide1/1
  Divide1/1 -> Add3/2
  Add3/1 -> PWM_us/1

== system DBX_Control_lib/Transl Eqs_ Get forces ==
  A_des : Inport
  Vb : Inport  Port=2
  omega_b : Inport  Port=3
  omega_b_dot : Inport  Port=4
  m : Inport  Port=5
  CG : Inport  Port=6
  Add : Sum  Inputs=++++
  Cross Product{,1..3} (4 alike) : vrlib/Utilities/Cross Product
  Product : Product  RndMeth=Zero
  Forces_des : Outport
  wires:
  Add/1 -> Product/1
  Cross Product/1 -> Add/3
  Cross Product3/1 -> Add/2
  Cross Product2/1 -> Add/1
  omega_b_dot/1 -> Cross Product3/1
  Cross Product1/1 -> Cross Product2/2
  CG/1 -> Cross Product1/2, Cross Product3/2
  Vb/1 -> Cross Product/2
  omega_b/1 -> Cross Product/1, Cross Product1/1, Cross Product2/1
  m/1 -> Product/2
  A_des/1 -> Add/4
  Product/1 -> Forces_des/1

== system DBX_Control_lib/2D vec norm/norm^2rm ==
  v : Inport
  Demux : Demux  Outputs=2
  Product : Product
  Product1 : Product
  Sum : Sum  Inputs=2
  norm(v) : Outport
  wires:
  v/1 -> Demux/1
  Sum/1 -> norm(v)/1
  Product/1 -> Sum/1
  Product1/1 -> Sum/2
  Demux/1 -> Product/1, Product/2
  Demux/2 -> Product1/2, Product1/1

== system DBX_Control_lib/3D vec norm/norm^2rm ==
  v : Inport
  Demux : Demux  Outputs=3
  Product : Product
  Product1 : Product
  Product2 : Product
  Sum : Sum  Inputs=3
  norm(v) : Outport
  wires:
  Demux/2 -> Product1/2, Product1/1
  Demux/1 -> Product/2, Product/1
  Product1/1 -> Sum/2
  Product/1 -> Sum/1
  Sum/1 -> norm(v)/1
  v/1 -> Demux/1
  Demux/3 -> Product2/2, Product2/1
  Product2/1 -> Sum/3

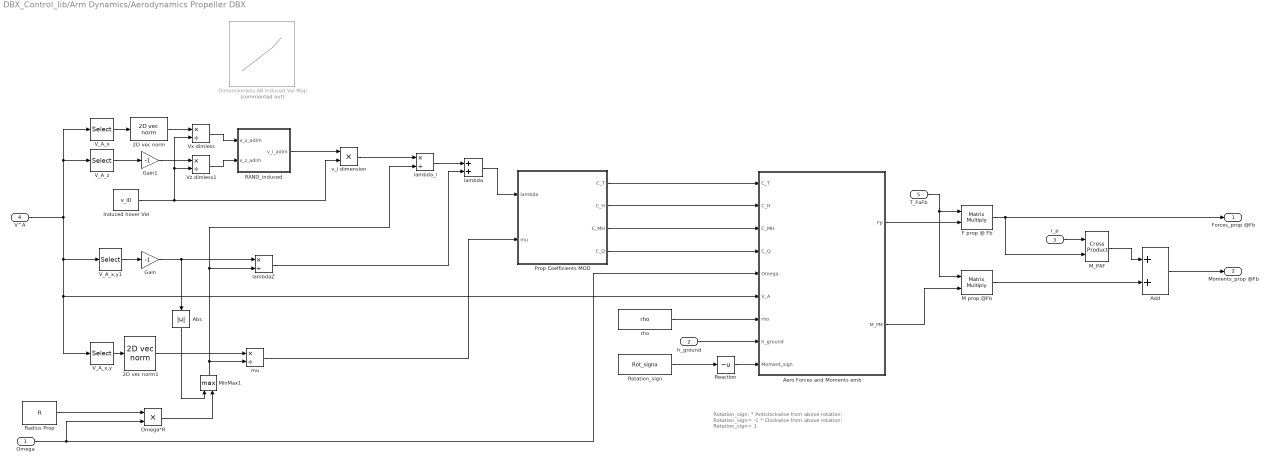
== system DBX_Control_lib/Arm Dynamics/Aerodynamics Propeller DBX ==
  note: Rotation_sign:
      |
      | * Anticlockwise from above rotation: Rotation_sign= -1
      | * Clockwise from above rotation: Rotation_sign= 1
  Omega : Inport
  h_ground : Inport  Port=2
  r_p : Inport  Port=3
  V^A : Inport  Port=4
  T_FaFb : Inport  Port=5
  2D vec norm : DBX_model/2D vec norm
  2D vec norm1 : DBX_model/2D vec norm
  Abs : Abs
  Add : Sum
  Aero Forces and Moments emb : Subsystem  TreatAsAtomicUnit=on
  Dimensionless AB induced Vel Map : Lookup_n-D  Commented=on  BreakpointsForDimension1=Vx_adim  BreakpointsForDimension2=Vz_adim  BreakpointsForDimension3=[5, 7]  Table=v_i_adim  RndMeth=Simplest  InputSameDT=on
  F prop @ Fb : Product  Multiplication=Matrix(*)
  Gain : Gain  Gain=-1
  Gain1 : Gain  Gain=-1
  Induced hover Vel : Constant  Value=v_i0  OutDataTypeStr=single
  M prop @Fb : Product  Multiplication=Matrix(*)
  M_PAF : vrlib/Utilities/Cross Product
  MinMax1 : MinMax  Function=max  Inputs=2
  Omega*R : Product  Inputs=**
  Prop Coefficients MOD : MATLAB Function  TreatAsAtomicUnit=on
  RAND_induced : Subsystem
  Radius Prop : Constant  Value=R  OutDataTypeStr=single
  Reaction : UnaryMinus
  Rotation_sign : Constant  Value=Rot_signa  OutDataTypeStr=single
  V_A_x : Selector  InputPortWidth=3  Indices=[1 2]
  V_A_x,y : Selector  InputPortWidth=3  Indices=[1 2]
  V_A_x,y1 : Selector  InputPortWidth=3  Indices=[3]
  V_A_z : Selector  InputPortWidth=3  Indices=3
  Vx dimless : Product  Inputs=*/
  Vz dimless1 : Product  Inputs=*/
  lambda : Sum
  lambdaZ : Product  Inputs=*/
  lambda_i : Product  Inputs=*/
  mu : Product  Inputs=*/
  rho : Constant  Value=rho  OutDataTypeStr=single
  v_i dimension : Product  Inputs=**
  Forces_prop @Fb : Outport
  Moments_prop @Fb : Outport  Port=2
  wires:
  Aero Forces and Moments emb/2("M_PM ") -> M prop @Fb/2
  Omega/1 -> Omega*R/2, Aero Forces and Moments emb/5(Omega)
  Omega*R/1 -> MinMax1/2
  Abs/1 -> MinMax1/1
  MinMax1/1 -> lambda_i/2, lambdaZ/2, mu/2
  rho/1 -> Aero Forces and Moments emb/7(rho)
  Reaction/1 -> Aero Forces and Moments emb/9(Moment_sign)
  Prop Coefficients MOD/4(C_Q) -> Aero Forces and Moments emb/4(C_Q)
  mu/1 -> Prop Coefficients MOD/2(mu)
  2D vec norm/1 -> Vx dimless/1
  M prop @Fb/1 -> Add/2
  M_PAF/1 -> Add/1
  r_p/1 -> M_PAF/1
  F prop @ Fb/1 -> Forces_prop @Fb/1, M_PAF/2
  Aero Forces and Moments emb/1(Fp) -> F prop @ Fb/2
  T_FaFb/1 -> F prop @ Fb/1, M prop @Fb/1
  Rotation_sign/1 -> Reaction/1
  h_ground/1 -> Aero Forces and Moments emb/8(h_ground)
  Add/1 -> Moments_prop @Fb/1
  V^A/1 -> V_A_z/1, V_A_x/1, V_A_x,y1/1, Aero Forces and Moments emb/6(V_A), V_A_x,y/1
  Prop Coefficients MOD/3(C_MH) -> Aero Forces and Moments emb/3(C_MH)
  Prop Coefficients MOD/2(C_H) -> Aero Forces and Moments emb/2(C_H)
  Prop Coefficients MOD/1(C_T) -> Aero Forces and Moments emb/1(C_T)
  lambda/1 -> Prop Coefficients MOD/1(lambda)
  Gain1/1 -> Vz dimless1/1
  lambdaZ/1 -> lambda/2
  lambda_i/1 -> lambda/1
  Gain/1 -> Abs/1, lambdaZ/1
  V_A_x,y1/1 -> Gain/1
  v_i dimension/1 -> lambda_i/1
  RAND_induced/1(v_i_adim) -> v_i dimension/1
  Induced hover Vel/1 -> Vx dimless/2, Vz dimless1/2, v_i dimension/2
  V_A_z/1 -> Gain1/1
  Vz dimless1/1 -> RAND_induced/2(v_z_adim)
  V_A_x/1 -> 2D vec norm/1
  Vx dimless/1 -> RAND_induced/1(v_x_adim)
  2D vec norm1/1 -> mu/1
  V_A_x,y/1 -> 2D vec norm1/1
  Radius Prop/1 -> Omega*R/1

== system DBX_Control_lib/Arm Dynamics/Arms Kinematics DBX ==
  eta (rad) : Inport
  Add3 : Sum
  Arm_no : Constant  Value=Value  OutDataTypeStr=single
  DCM Arm : MATLAB Function  TreatAsAtomicUnit=on
  Fa->Fb : Product  Multiplication=Matrix(*)
  Gain7 : Gain  Gain=[0;0;1]  OutDataTypeStr=single
  Hub_position aka r_RP_i : Constant  Value=Hub_pos  OutDataTypeStr=single
  Permute Dimensions : PermuteDimensions
  h_p_i : Constant  Value=h_p  OutDataTypeStr=single
  r_p (m) : Outport
  T_F_a,Fb : Outport  Port=2
  wires:
  DCM Arm/1(T_Fb_FA) -> Permute Dimensions/1
  Permute Dimensions/1 -> T_F_a,Fb/1, Fa->Fb/1  "T_F_a,Fb"
  eta (rad)/1 -> DCM Arm/2(eta)
  Add3/1 -> r_p (m)/1  "r_p (m)"
  h_p_i/1 -> Gain7/1
  Gain7/1 -> Fa->Fb/2
  Hub_position aka r_RP_i/1 -> Add3/1
  Fa->Fb/1 -> Add3/2
  Arm_no/1 -> DCM Arm/1(arm_no)

== system DBX_Control_lib/Arm Dynamics/ESC+Motor Dynamcis  ==
  Throttle : Inport
  2-D Throtle-Omega curve : Fcn  Expr=-45.2192+43.046*u(1)-1.21*u(1)^2+0.0144*u(1)^3
  2-D Throttle-Omega Map : Lookup_n-D  Commented=on  NumberOfTableDimensions=1  BreakpointsForDimension1=Throtle_TO  BreakpointsForDimension2=Throtle_TTO_vec  Table=Omega_TO  TableDataTypeStr=single  IntermediateResultsDataTypeStr=single  ExtrapMethod=Clip  DiagnosticForOutOfRangeInput=Warning  RemoveProtectionInput=on  OutDataTypeStr=single  RndMeth=Zero  FractionDataTypeStr=single  InputSameDT=on
  Bias : Bias  Bias=eps
  Omega_out : Outport
  wires:
  2-D Throtle-Omega curve/1 -> Bias/1
  Bias/1 -> Omega_out/1
  Throttle/1 -> 2-D Throtle-Omega curve/1

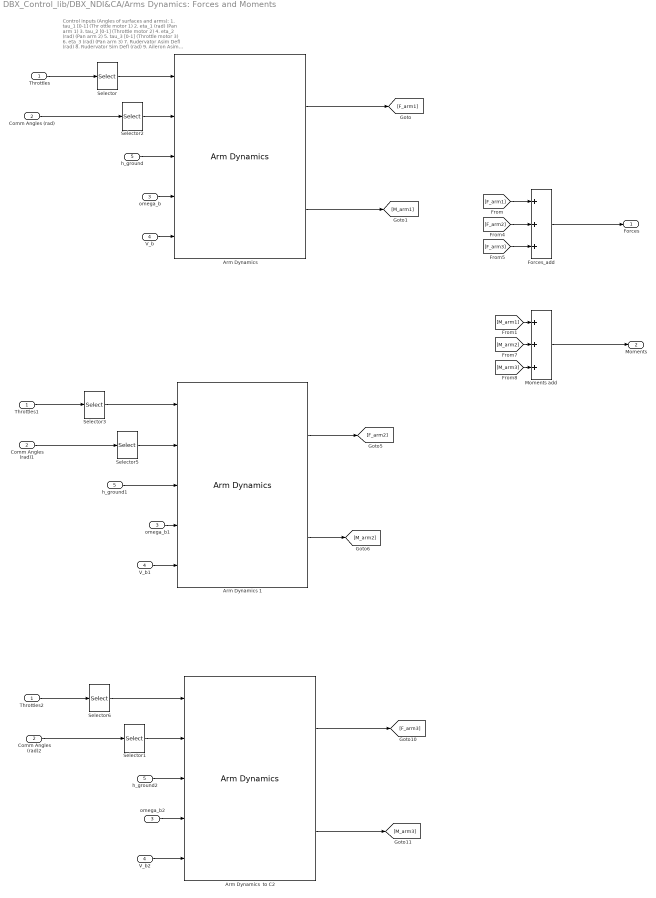
== system DBX_Control_lib/DBX_NDI&CA/Arms Dynamics: Forces and Moments ==
  note: Control inputs (Angles  of surfaces and arms):
      |
      | 1. tau_1 [0-1] (Thr ottle motor 1)
      | 2. eta_1 (rad)  (Pan arm 1)
      |
      | 3. tau_2 [0-1] (Throttle motor 2)
      | 4. eta_2 (rad)  (Pan arm 2)
      |
      | 5. tau_3 [0-1] (Throttle motor 3)
      | 6. eta_3 (rad)  (Pan arm  3)
      |
      | 7. Rudervator Asim Defl (rad)
      | 8. Rudervator Sim Defl (rad)
      | 9. Aileron Asim Defl (rad)
  Throttles : Inport
  Comm Angles (rad) : Inport  Port=2
  omega_b : Inport  Port=3
  V_b : Inport  Port=4
  h_ground : Inport  Port=5
  "Arm Dynamics " : DBX_Control_lib/Arm Dynamics  arm_num=1  Rot_sign=Rotation_sign(1)  Hub_pos=[1/3*L_M;-A_M/2;h_1]  h_p=hp_1
  Arm Dynamics  to C2 : DBX_Control_lib/Arm Dynamics  arm_num=3  Rot_sign=Rotation_sign(3)  Hub_pos=[-2/3*L_M;0;h_3]  h_p=hp_3
  Arm Dynamics 1 : DBX_Control_lib/Arm Dynamics  arm_num=2  Rot_sign=Rotation_sign(2)  Hub_pos=[1/3*L_M;A_M/2;h_2]  h_p=hp_2
  Comm Angles (rad)1 : InportShadow  Port=2
  Comm Angles (rad)2 : InportShadow  Port=2
  Forces_add : Sum  Inputs=+++
  Moments add : Sum  Inputs=+++
  Selector : Selector  IndexMode=Zero-based  InputPortWidth=3  Indices=0
  Selector1 : Selector  IndexMode=Zero-based  InputPortWidth=3  Indices=2
  Selector2 : Selector  InputPortWidth=3
  Selector3 : Selector  IndexMode=Zero-based  InputPortWidth=3
  Selector5 : Selector  InputPortWidth=3  Indices=2
  Selector6 : Selector  IndexMode=Zero-based  InputPortWidth=3  Indices=2
  Throttles1 : InportShadow
  Throttles2 : InportShadow
  V_b1 : InportShadow  Port=4
  V_b2 : InportShadow  Port=4
  h_ground1 : InportShadow  Port=5
  h_ground2 : InportShadow  Port=5
  omega_b1 : InportShadow  Port=3
  omega_b2 : InportShadow  Port=3
  Forces : Outport
  Moments : Outport  Port=2
  wires:
  V_b2/1 -> Arm Dynamics  to C2/5
  Arm Dynamics 1/2 -> [M_arm2]
  Throttles/1 -> Selector/1
  Selector/1 -> "Arm Dynamics "/1
  V_b/1 -> "Arm Dynamics "/5
  Forces_add/1 -> Forces/1
  Moments add/1 -> Moments/1
  h_ground/1 -> "Arm Dynamics "/3
  "Arm Dynamics "/1 -> [F_arm1]
  "Arm Dynamics "/2 -> [M_arm1]
  [F_arm1] -> Forces_add/1
  [M_arm1] -> Moments add/1
  omega_b/1 -> "Arm Dynamics "/4
  [F_arm2] -> Forces_add/2
  [F_arm3] -> Forces_add/3
  [M_arm3] -> Moments add/3
  [M_arm2] -> Moments add/2
  Selector2/1 -> "Arm Dynamics "/2
  Comm Angles (rad)/1 -> Selector2/1
  Throttles1/1 -> Selector3/1
  Selector3/1 -> Arm Dynamics 1/1
  V_b1/1 -> Arm Dynamics 1/5
  h_ground1/1 -> Arm Dynamics 1/3
  omega_b1/1 -> Arm Dynamics 1/4
  Selector5/1 -> Arm Dynamics 1/2
  Comm Angles (rad)1/1 -> Selector5/1
  Throttles2/1 -> Selector6/1
  Selector6/1 -> Arm Dynamics  to C2/1
  h_ground2/1 -> Arm Dynamics  to C2/3
  Arm Dynamics  to C2/1 -> [F_arm3]
  Arm Dynamics  to C2/2 -> [M_arm3]
  omega_b2/1 -> Arm Dynamics  to C2/4
  Selector1/1 -> Arm Dynamics  to C2/2
  Comm Angles (rad)2/1 -> Selector1/1
  Arm Dynamics 1/1 -> [F_arm2]

== system DBX_Control_lib/DBX_NDI&CA/Gradient of arms contributions (1:6) ==
  note: Control inputs (Angles  of surfaces and arms):
      |
      | 1. tau_1 [0-1] (Thr ottle motor 1)
      | 2. eta_1 (rad)  (Pan arm 1)
      |
      | 3. tau_2 [0-1] (Throttle motor 2)
      | 4. eta_2 (rad)  (Pan arm 2)
      |
      | 5. tau_3 [0-1] (Throttle motor 3)
      | 6. eta_3 (rad)  (Pan arm  3)
      |
      | 7. Rudervator Asim Defl (rad)
      | 8. Rudervator Sim Defl (rad)
      | 9. Aileron Asim Defl (rad)
  Curr_V : Inport  Partition=off
  "Control Inputs(rad) " : Inport  Port=2  Partition=on  PartitionDimension=1  PartitionWidth=6
  h : Inport  Port=3  Partition=off
  Vb : Inport  Port=4  Partition=off
  omega_b : Inport  Port=5  Partition=off
  F_g : Inport  Port=6  Partition=off
  M_g : Inport  Port=7  Partition=off
  Add : Sum
  Add1 : Sum
  Arms Dynamics: Forces and Moments : Subsystem  TreatAsAtomicUnit=on
  Equivalent Throttle : Product  Inputs=**
  For Each : ForEach  DisableCoverage=on  IndexMode=One-based
  Mux : Mux  Inputs=[3,3]
  Signal Specification : SignalSpecification  Dimensions=[6,1]
  Throttles : Selector  InputPortWidth=6  Indices=[1,3,5]
  "angles " : Selector  InputPortWidth=6  Indices=[2,4,6]
  Forces_Moments : Outport  ConcatenationDimension=2
  wires:
  Vb/1 -> Arms Dynamics: Forces and Moments/4(V_b)
  Arms Dynamics: Forces and Moments/2(Moments) -> Add1/1
  "angles "/1 -> Arms Dynamics: Forces and Moments/2(Comm Angles (rad))
  omega_b/1 -> Arms Dynamics: Forces and Moments/3(omega_b)
  h/1 -> Arms Dynamics: Forces and Moments/5(h_ground)
  Arms Dynamics: Forces and Moments/1(Forces) -> Add/1
  Throttles/1 -> Equivalent Throttle/2
  "Control Inputs(rad) "/1 -> Throttles/1, "angles "/1
  Equivalent Throttle/1 -> Arms Dynamics: Forces and Moments/1(Throttles)
  Curr_V/1 -> Equivalent Throttle/1
  F_g/1 -> Add/2
  M_g/1 -> Add1/2
  Add/1 -> Mux/1
  Add1/1 -> Mux/2
  Mux/1 -> Signal Specification/1
  Signal Specification/1 -> Forces_Moments/1

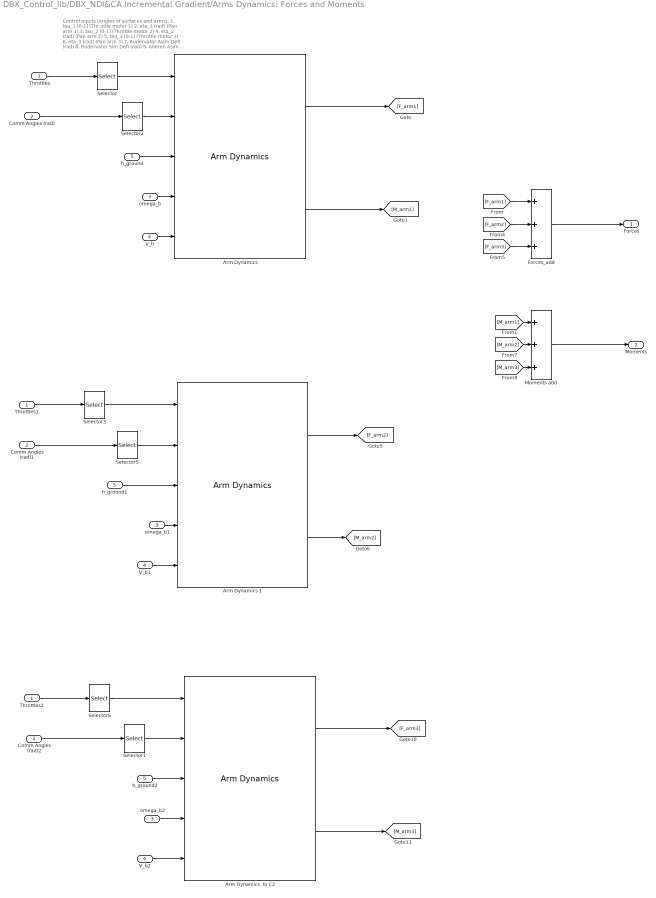
== system DBX_Control_lib/DBX_NDI&CA Incremental Gradient/Arms Dynamics: Forces and Moments ==
  note: Control inputs (Angles  of surfaces and arms):
      |
      | 1. tau_1 [0-1] (Thr ottle motor 1)
      | 2. eta_1 (rad)  (Pan arm 1)
      |
      | 3. tau_2 [0-1] (Throttle motor 2)
      | 4. eta_2 (rad)  (Pan arm 2)
      |
      | 5. tau_3 [0-1] (Throttle motor 3)
      | 6. eta_3 (rad)  (Pan arm  3)
      |
      | 7. Rudervator Asim Defl (rad)
      | 8. Rudervator Sim Defl (rad)
      | 9. Aileron Asim Defl (rad)
  Throttles : Inport
  Comm Angles (rad) : Inport  Port=2
  omega_b : Inport  Port=3
  V_b : Inport  Port=4
  h_ground : Inport  Port=5
  "Arm Dynamics " : DBX_Control_lib/Arm Dynamics  arm_num=1  Rot_sign=Rotation_sign(1)  Hub_pos=[1/3*L_M;-A_M/2;h_1]  h_p=hp_1
  Arm Dynamics  to C2 : DBX_Control_lib/Arm Dynamics  arm_num=3  Rot_sign=Rotation_sign(3)  Hub_pos=[-2/3*L_M;0;h_3]  h_p=hp_3
  Arm Dynamics 1 : DBX_Control_lib/Arm Dynamics  arm_num=2  Rot_sign=Rotation_sign(2)  Hub_pos=[1/3*L_M;A_M/2;h_2]  h_p=hp_2
  Comm Angles (rad)1 : InportShadow  Port=2
  Comm Angles (rad)2 : InportShadow  Port=2
  Forces_add : Sum  Inputs=+++
  Moments add : Sum  Inputs=+++
  Selector : Selector  IndexMode=Zero-based  InputPortWidth=3  Indices=0
  Selector1 : Selector  IndexMode=Zero-based  InputPortWidth=3  Indices=2
  Selector2 : Selector  InputPortWidth=3
  Selector3 : Selector  IndexMode=Zero-based  InputPortWidth=3
  Selector5 : Selector  InputPortWidth=3  Indices=2
  Selector6 : Selector  IndexMode=Zero-based  InputPortWidth=3  Indices=2
  Throttles1 : InportShadow
  Throttles2 : InportShadow
  V_b1 : InportShadow  Port=4
  V_b2 : InportShadow  Port=4
  h_ground1 : InportShadow  Port=5
  h_ground2 : InportShadow  Port=5
  omega_b1 : InportShadow  Port=3
  omega_b2 : InportShadow  Port=3
  Forces : Outport
  Moments : Outport  Port=2
  wires:
  V_b2/1 -> Arm Dynamics  to C2/5
  Arm Dynamics 1/2 -> [M_arm2]
  Throttles/1 -> Selector/1
  Selector/1 -> "Arm Dynamics "/1
  V_b/1 -> "Arm Dynamics "/5
  Forces_add/1 -> Forces/1
  Moments add/1 -> Moments/1
  h_ground/1 -> "Arm Dynamics "/3
  "Arm Dynamics "/1 -> [F_arm1]
  "Arm Dynamics "/2 -> [M_arm1]
  [F_arm1] -> Forces_add/1
  [M_arm1] -> Moments add/1
  omega_b/1 -> "Arm Dynamics "/4
  [F_arm2] -> Forces_add/2
  [F_arm3] -> Forces_add/3
  [M_arm3] -> Moments add/3
  [M_arm2] -> Moments add/2
  Selector2/1 -> "Arm Dynamics "/2
  Comm Angles (rad)/1 -> Selector2/1
  Throttles1/1 -> Selector3/1
  Selector3/1 -> Arm Dynamics 1/1
  V_b1/1 -> Arm Dynamics 1/5
  h_ground1/1 -> Arm Dynamics 1/3
  omega_b1/1 -> Arm Dynamics 1/4
  Selector5/1 -> Arm Dynamics 1/2
  Comm Angles (rad)1/1 -> Selector5/1
  Throttles2/1 -> Selector6/1
  Selector6/1 -> Arm Dynamics  to C2/1
  h_ground2/1 -> Arm Dynamics  to C2/3
  Arm Dynamics  to C2/1 -> [F_arm3]
  Arm Dynamics  to C2/2 -> [M_arm3]
  omega_b2/1 -> Arm Dynamics  to C2/4
  Selector1/1 -> Arm Dynamics  to C2/2
  Comm Angles (rad)2/1 -> Selector1/1
  Arm Dynamics 1/1 -> [F_arm2]

== system DBX_Control_lib/DBX_NDI&CA Incremental Gradient/Gradient of arms contributions (1:6) ==
  note: Control inputs (Angles  of surfaces and arms):
      |
      | 1. tau_1 [0-1] (Thr ottle motor 1)
      | 2. eta_1 (rad)  (Pan arm 1)
      |
      | 3. tau_2 [0-1] (Throttle motor 2)
      | 4. eta_2 (rad)  (Pan arm 2)
      |
      | 5. tau_3 [0-1] (Throttle motor 3)
      | 6. eta_3 (rad)  (Pan arm  3)
      |
      | 7. Rudervator Asim Defl (rad)
      | 8. Rudervator Sim Defl (rad)
      | 9. Aileron Asim Defl (rad)
  Curr_V : Inport  Partition=off
  "Control Inputs(rad) " : Inport  Port=2  Partition=on  PartitionDimension=1  PartitionWidth=6
  h : Inport  Port=3  Partition=off
  Vb : Inport  Port=4  Partition=off
  omega_b : Inport  Port=5  Partition=off
  F_g : Inport  Port=6  Partition=off
  M_g : Inport  Port=7  Partition=off
  Add : Sum
  Add1 : Sum
  Arms Dynamics: Forces and Moments : Subsystem  TreatAsAtomicUnit=on
  Equivalent Throttle : Product  Inputs=**
  For Each : ForEach  DisableCoverage=on  IndexMode=One-based
  Mux : Mux  Inputs=[3,3]
  Signal Specification : SignalSpecification  Dimensions=[6,1]
  Throttles : Selector  InputPortWidth=6  Indices=[1,3,5]
  "angles " : Selector  InputPortWidth=6  Indices=[2,4,6]
  Forces_Moments : Outport  ConcatenationDimension=2
  wires:
  Vb/1 -> Arms Dynamics: Forces and Moments/4(V_b)
  Arms Dynamics: Forces and Moments/2(Moments) -> Add1/1
  "angles "/1 -> Arms Dynamics: Forces and Moments/2(Comm Angles (rad))
  omega_b/1 -> Arms Dynamics: Forces and Moments/3(omega_b)
  h/1 -> Arms Dynamics: Forces and Moments/5(h_ground)
  Arms Dynamics: Forces and Moments/1(Forces) -> Add/1
  Throttles/1 -> Equivalent Throttle/2
  "Control Inputs(rad) "/1 -> Throttles/1, "angles "/1
  Equivalent Throttle/1 -> Arms Dynamics: Forces and Moments/1(Throttles)
  Curr_V/1 -> Equivalent Throttle/1
  F_g/1 -> Add/2
  M_g/1 -> Add1/2
  Add/1 -> Mux/1
  Add1/1 -> Mux/2
  Mux/1 -> Signal Specification/1
  Signal Specification/1 -> Forces_Moments/1

== system DBX_Control_lib/GCS params safemode/Sample&Hold ==
  In1 : Inport
  Trigger : TriggerPort
  Out1 : Outport
  wires:
  In1/1 -> Out1/1

== system DBX_Control_lib/Normalize 4D vector/4D vec norm ==
  v : Inport
  norm^2rm : Subsystem  TreatAsAtomicUnit=on
  sqrt : Sqrt  AlgorithmType=Newton-Raphson  SaturateOnIntegerOverflow=on
  norm(v) : Outport
  wires:
  sqrt/1 -> norm(v)/1
  norm^2rm/1(norm(v)) -> sqrt/1
  v/1 -> norm^2rm/1(v)
